simulink model "Project_model"  (R2016b)
settings: Solver=VariableStepAuto  StartTime=0.0  StopTime=10.0  RelTol=1e-3
values from neighbouring files (symbols this model uses):
  b = 0    [Project_param.m]
  J = 2.7e-7    (= 2.7e-07)    [Project_param.m]
  K = 11.12e-3    (= 0.01112)    [Project_param.m]
  L = 130e-6    (= 0.00013)    [Project_param.m]
  l = 0.12    [Project_param.m]
  R = 10    [Project_param.m]
  r = 0.065    [Project_param.m]
settings Model: Creator=Philip  LastModifiedBy=Philip

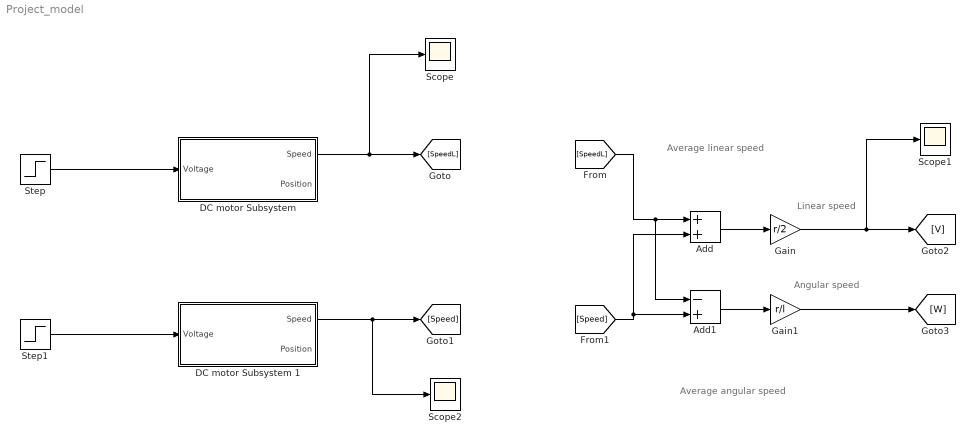
== system Project_model ==
  note: Average angular speed
  note: Average linear speed
  note: Angular speed
  note: Linear speed
  Add : Sum
  Add1 : Sum  Inputs=-+
  "DC motor Subsystem " : Subsystem
  DC motor Subsystem 1 : Subsystem
  Gain : Gain  Gain=r/2
  Gain1 : Gain  Gain=r/l
  Scope : Scope
  Scope1 : Scope
  Scope2 : Scope
  Step : Step  Time=0.1  After=8  SampleTime=0
  Step1 : Step  Time=0.1  After=5  SampleTime=0
  wires:
  Step/1 -> "DC motor Subsystem "/1("Voltage ")
  Step1/1 -> DC motor Subsystem 1/1("Voltage ")
  DC motor Subsystem 1/1("Speed ") -> Scope2/1, [Speed]
  [Speed] -> Add1/2, Add/2
  [SpeedL] -> Add1/1, Add/1
  Add/1 -> Gain/1
  Gain/1 -> Scope1/1, [V]
  Add1/1 -> Gain1/1
  Gain1/1 -> [W]
  "DC motor Subsystem "/1("Speed ") -> Scope/1, [SpeedL]

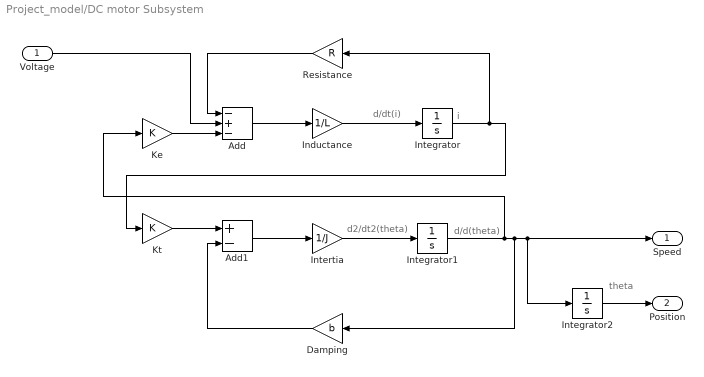
== system Project_model/DC motor Subsystem  ==
  note: theta
  note: d/dt(i)
  note: i
  note: d/d(theta)
  note: d2/dt2(theta)
  "Voltage " : Inport
  Add : Sum  Inputs=-+-
  Add1 : Sum  Inputs=+-
  "Damping " : Gain  Gain=b
  "Inductance " : Gain  Gain=1/L
  Integrator : Integrator
  Integrator1 : Integrator
  Integrator2 : Integrator
  "Intertia " : Gain  Gain=1/J
  Ke : Gain  Gain=K
  "Kt " : Gain  Gain=K
  "Resistance " : Gain  Gain=R
  "Speed " : Outport
  "Position " : Outport  Port=2
  wires:
  Integrator/1 -> "Resistance "/1, "Kt "/1
  Add1/1 -> "Intertia "/1
  Integrator1/1 -> Ke/1, Integrator2/1, "Speed "/1, "Damping "/1
  "Resistance "/1 -> Add/1
  "Voltage "/1 -> Add/2
  Ke/1 -> Add/3
  Add/1 -> "Inductance "/1
  "Intertia "/1 -> Integrator1/1
  "Inductance "/1 -> Integrator/1
  "Damping "/1 -> Add1/2
  "Kt "/1 -> Add1/1
  Integrator2/1 -> "Position "/1

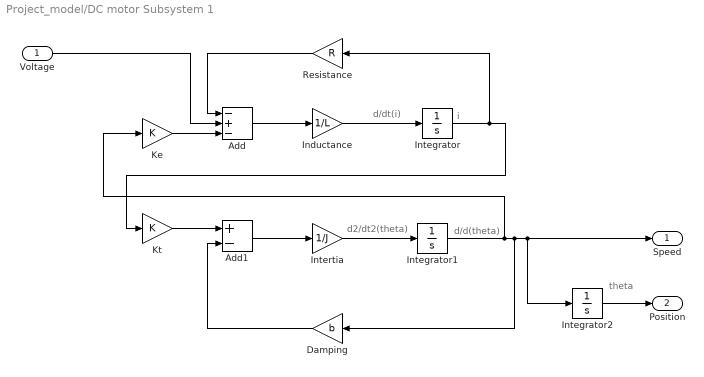
== system Project_model/DC motor Subsystem 1 ==
  note: theta
  note: d/dt(i)
  note: i
  note: d/d(theta)
  note: d2/dt2(theta)
  "Voltage " : Inport
  Add : Sum  Inputs=-+-
  Add1 : Sum  Inputs=+-
  "Damping " : Gain  Gain=b
  "Inductance " : Gain  Gain=1/L
  Integrator : Integrator
  Integrator1 : Integrator
  Integrator2 : Integrator
  "Intertia " : Gain  Gain=1/J
  Ke : Gain  Gain=K
  "Kt " : Gain  Gain=K
  "Resistance " : Gain  Gain=R
  "Speed " : Outport
  "Position " : Outport  Port=2
  wires:
  Integrator/1 -> "Resistance "/1, "Kt "/1
  Add1/1 -> "Intertia "/1
  Integrator1/1 -> Ke/1, Integrator2/1, "Speed "/1, "Damping "/1
  "Resistance "/1 -> Add/1
  "Voltage "/1 -> Add/2
  Ke/1 -> Add/3
  Add/1 -> "Inductance "/1
  "Intertia "/1 -> Integrator1/1
  "Inductance "/1 -> Integrator/1
  "Damping "/1 -> Add1/2
  "Kt "/1 -> Add1/1
  Integrator2/1 -> "Position "/1
